simulink model "realtime_open_loop_test"  (R2018a)
settings: Solver=FixedStepAuto  StartTime=0.0  StopTime=inf  FixedStep=0.01  RelTol=1e-3
undefined symbols (not defined in the file): CR, LF, serial
libraries: instrumentlib x3, simulink x1
settings Model: Creator=Hp2  LastModifiedBy=Hp2

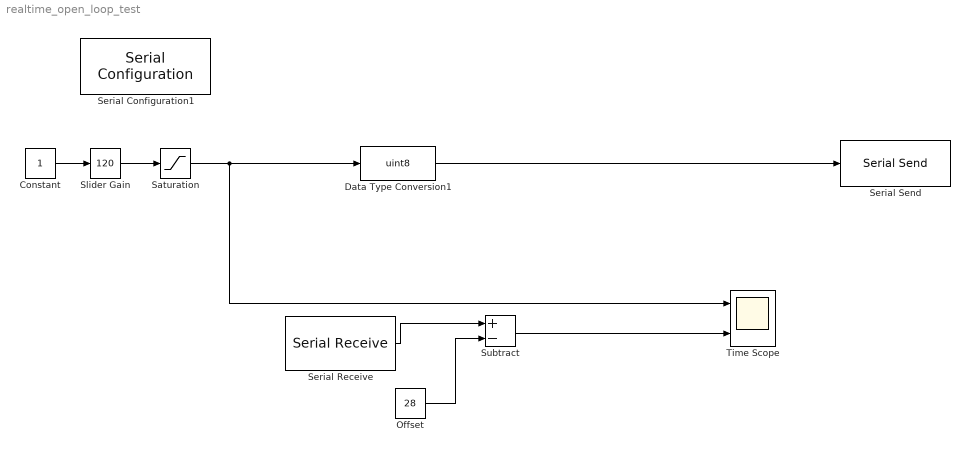
== system realtime_open_loop_test ==
  Constant : Constant  OutDataTypeStr=uint16  SampleTime=-1
  Data Type Conversion1 : DataTypeConversion  OutDataTypeStr=uint8
  Offset : Constant  Value=28  OutDataTypeStr=uint16  SampleTime=0.01
  Saturation : Saturate  UpperLimit=255  LowerLimit=1
  Serial Configuration1 : instrumentlib/Serial Configuration  Priority=-200000  ComPortMenu=COM6  ComPort=COM6  ObjConstructor=serial('COM6');  BaudRate=19200  DataBits=8  Parity=none  StopBits=1  FlowControl=none  Timeout=10  ByteOrder=LittleEndian
  Serial Receive : instrumentlib/Serial Receive  ComPortMenu=COM6  ComPort=COM6  ObjConstructor=serial('COM6');  Terminator=CR/LF ('\r\n')  DataSize=1  DataType=uint16  EnableBlockingMode=on  ActionDataUnavailable=Output last received value  CustomValue=0  SampleTime=-1
  Serial Send : instrumentlib/Serial Send  ComPortMenu=<Please select a port...>  ComPort=COM6  ObjConstructor=serial('COM6');  Terminator=<none>  EnableBlockingMode=off
  Slider Gain : simulink/Math Operations/Slider Gain  gain=120  low=1  high=1000
  Subtract : Sum  Inputs=+-  OutDataTypeStr=int16
  Time Scope : Scope  NumInputPorts=2
  wires:
  Data Type Conversion1/1 -> Serial Send/1
  Saturation/1 -> Time Scope/1, Data Type Conversion1/1
  Constant/1 -> Slider Gain/1
  Serial Receive/1 -> Subtract/1
  Slider Gain/1 -> Saturation/1
  Offset/1 -> Subtract/2
  Subtract/1 -> Time Scope/2
